simulink model "SF5_2_4_jc0531_2_B"  (R2016b)
settings: Solver=VariableStepAuto  StartTime=0.0  StopTime=inf  RelTol=1e-3  EnableMultiTasking=on
settings Model: Creator=amyyang  LastModifiedBy=amyyang
settings DataIOCC: LimitDataPoints=on
settings OptimizationCC: LifeSpan=inf
settings DebuggingCC: AllowSymbolicDim=off  SFUnexpectedBacktrackingDiag=warning  SFNoUnconditionalDefaultTransitionDiag=warning  SFExecutionAtInitializationDiag=none
settings ModelReferenceCC: PropagateSignalLabelsOutOfModel=off
settings GRTTargetCC: TargetLangStandard=C89/C90 (ANSI)
settings ConfigComp: CovMetricSettings=dw  CovHtmlReporting=on  CovSaveCumulativeToWorkspaceVar=on  CovSaveSingleToWorkspaceVar=on  CovExternalEMLEnable=off

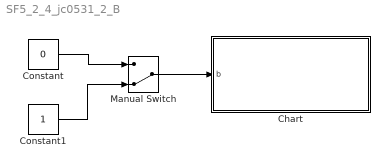
== system SF5_2_4_jc0531_2_B ==
  Chart : Stateflow chart  TreatAsAtomicUnit=on
  Constant : Constant  Value=0
  Constant1 : Constant
  Manual Switch : ManualSwitch  CurrentSetting=0
  wires:
  Manual Switch/1 -> Chart/1(b)
  Constant1/1 -> Manual Switch/2
  Constant/1 -> Manual Switch/1

== stateflow chart SF5_2_4_jc0531_2_B/Chart ==
  state B
    state BB1
    state BB2
    (default) -> BB1 [order 1]
    BB1 -> BB2 : after(5,sec)
    BB2 -> BB1 : after(5,sec)
    (default) -> BB2 [order 2]
  state A
  (default) -> A
  A -> B : [ b > 0]
  data: b input
